simulink model "plant_neural"  (R2020a)
settings: Solver=VariableStepAuto  StartTime=0.0  StopTime=200  RelTol=1e-3
values from neighbouring files (symbols this model uses):
  Ca = 0.005    [reproduce_examples.m]
  Cb = 0.005    [reproduce_examples.m]
  dt = 0.05    [reproduce_examples.m]
  fA = 2    [reproduce_examples.m]
  fB = 2    [reproduce_examples.m]
  V = 3    [reproduce_examples.m]
libraries: simulink x2, neural x1
settings Model: Creator=salvatore  LastModifiedBy=salvatore
settings DataIOCC: ExternalInput=Fb  FinalStateName=p  SaveFormat=Array  SignalLogging=off  OutputSaveName=pH, valve
settings DebuggingCC: UnderSpecifiedDimensionMsg=warning

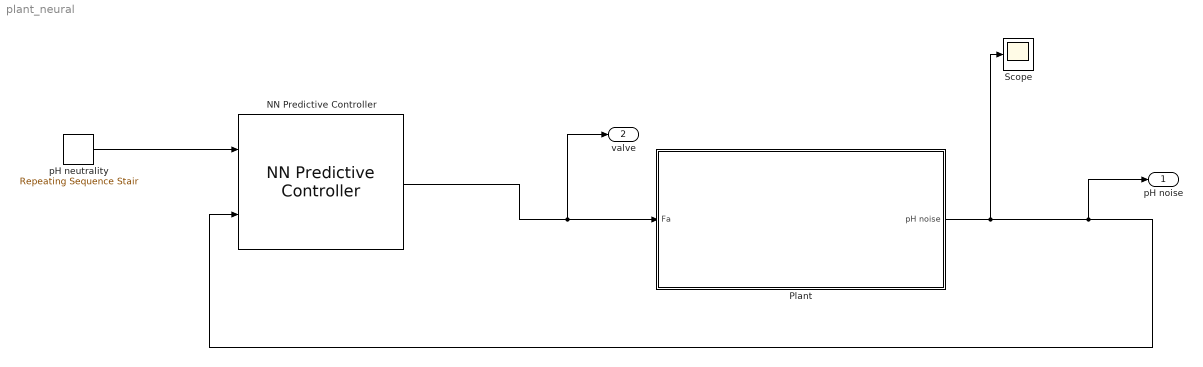
== system plant_neural ==
  NN Predictive Controller : neural/Control Systems/NN Predictive Controller  epochs=3000  minp=49.141375352717240332  maxp=50.989811034304850068  mint=4.3097489678251754697  maxt=50.989811034304850068  Normalize=0  IW=[-0.93780239581817526062 -0.66326789240486860866 -1.2871031244271990968;1.9683728574995722482 1.0271333939241629185 0.44317348386700522456;0.75017590865152150581 -1.0780019808511700496 1.0869414820155824941;1.4559030881353915987 -0.12800319720607680751 0.95276790366173158553;18.087212465487294111 -2.91864184413527461 -14.566729179573659536;1.2400378014953861161 0.1375233693964867665 0.77502847574575350897;0.33253977855035904421 1.7304982921477456426 1.3544701109704289088;0.64182775575216644004 1.4117570112710189356 -0.65500462374746837302;1.0980139843273326594 1.4813102838210283618 -1.1355980615640355325;-1.8940112774775548221 -1.0242663724758558352 -1.1299048301245802062;1.855202007600092351 0.12165935101839298049 -0.79891607712896228755;-0.32930667884939862633 -1.5538501135001399067 -0.75067226960660971002;-1.072431998622664695 0.65403235548163929369 1.0984496057562562754;0.81019484569678412722 0.33526087379087021745 -1.5256456319409121836;-1.4522827265983397904 1.485812570700000057 0.37966236721378082697;-1.1923047419461934027 1.5162107446574706326 -1.0145022129936238642;0.30440125275836227292 1.3381364521867997741 1.0876416367064514201;-0.92200869750636560429 -0.32060881750568615001 -1.2246860483548469567;-0.60210950948219532641 -1.4986276837771175252 -0.080409026582326029176;-0.403355788115020375 0.24290872576269775807 2.3590303610904217457;-0.19706504822617046391 -1.023417972628119843 -0.52486522394001777769;-0.3686768376053149443 -0.88079531358954077369 -1.5303785213897103112;0.53120649011313425536 -0.82254467800489938778 -1.3528928606977603799;-1.2733849000756418679 -1.6495155478202192523 -0.39519231325363640694;-1.302693854262735762 1.0188200785665699755 -0.7030027146678801131;-1.3444294028268313212 0.92366281600611421787 -0.89920403196537579404;-0.71934229537864724513 0.098840184553247473209 1.9183675969502649306;1.1859515817055199527 -0.72039123611880495623 0.80635457452268266554;-0.91328157335381698889 1.1116547471258793056 1.5977262904151019463;0.88358410119703434393 0.18945012830566010376 -0.20403044228299269114;0.68771194682422021049 1.5767992308421543424 1.5215138710997695437;1.1746781130618693112 1.3205123690215239129 -1.7492648228398455235;1.366694751554343723 -0.59956811717985569743 0.46771085416193147744;-0.76196806167879460592 0.11135710623432852617 1.1872906506293119389;-0.63585738589058671266 -0.51021415961426375141 -0.93569241318754825532;0.15302930875759376828 0.38592558000686749686 1.4065606172366182935;-1.0258043101484959347 1.6494109276893627047 1.4700854999973029802;1.1035774350367175689 0.78663020300303343468 1.0269086353427672176;1.0614598671358197457 -1.2948141427555899252 0.25657285536884832933;0.048561450203500375333 1.1539886836612518461 1.0587047076348954366]  LW1_2=[-0.62041762781086506884 -1.2878921055441192589 1.3341064249686134247;-0.4452363508536192338 0.41776855322875938725 -0.16173792171746106949;0.7856277323655095346 -1.4328813778630613562 -1.4048068556256605444;-1.1026662378935343511 -0.13613422789046639161 -1.582104961796532594;9.2826822808918620922 -15.216546321325413516 1.746026347965279113;-0.89963594778431121846 -1.5624571017304575982 -1.1696900531712195459;-1.0380744821846603632 0.80818670706969764073 -0.28584295651548530248;-2.0100154521868383029 -2.7516072687074384362 1.5959436752205937715;1.1440492783128197729 0.83935914794030452857 0.13137238494993638827;-0.17328463839084443099 -0.30390637859945579535 -0.51995736605186482215;-0.54032173048821574568 -0.38414956417682477596 -1.3561814656743973462;-1.0874881996895870984 -1.5564886858033175621 -0.19773337940546048541;1.1710921340230626697 -1.0606306130658302855 1.1424339619712420291;-0.34790852481674128249 -1.3671355131979634479 -1.2360864438805858612;1.4392017742796474611 0.38518544750179245506 -0.12885364617398359366;0.41412038455630650891 -0.79867140581223539098 1.0466562009230124808;-0.42970303418967958908 1.0765221590345304126 -1.4956312828675100146;1.4379506574267850727 1.2978382988600296599 0.67962005247037582389;0.89538010453812910683 1.276425240546694706 1.3508334040361238415;-0.16637092117171603523 0.0048575864307608667553 -0.95787243818502754156;1.0941255058475363171 -1.2496437309479786482 -1.6035705320276094632;1.4249238601570537455 -0.95316005127912184491 0.63714090417240143438;-0.32080390345351345038 0.16230007420602191037 1.9459977888606936336;-0.66671428962549628139 1.134168699749920517 0.55528982774655066823;0.39914983905510748041 -0.60645365770087922286 1.7410306582268146869;1.369987504183791005 -0.17140586938442378684 -1.1112576424741043013;0.88535442154446764018 0.59339915818222865873 1.1636166105827401296;-0.51693099978261292105 1.8481114067055248729 -0.64860148033353415276;0.86149168240209295089 -1.1144179111944447769 -0.29601512276503749721;1.8168695740521629833 0.9606138608186394201 -1.2248969681246073549;0.18613707562859144184 0.31093738389837610736 1.1586827272944042466;0.18384056074634250177 -0.06569561361777594144 0.53337760519972754469;-0.79892203697135377727 1.6575502283018046512 0.97902857163499057425;-1.7227854292604303232 -0.46185913158445146554 1.2421345908758245624;-1.1699157231057202289 -1.1656192475389974827 -1.5771178680323889587;-1.3992694065135036219 0.36304775877899103653 1.551469629702085351;-0.19023048985576973546 0.7495605338521728056 0.036042435367489758513;-1.5862432648658111312 -0.51387741920938923013 0.93417374728402524653;1.4268590699500380836 1.0441978897072439203 0.83533526411353720142;0.47269246211427085047 1.4569527321962194577 0.90941043120806075439]  LW2_1=[-0.66653421186476879967 -2.3712304948727283005 0.11942670348945146064 0.30208230055944201853 -0.15692778228640197336 -0.35950126395863518658 0.09773454763742397966 -0.41867824898828193136 0.5537078005106340628 0.36924865693212843842 -0.38671729588311865022 0.38461463905337617275 0.47125947419330549426 -0.71456955098225838352 0.10753548983805111261 -0.3776052745659378429 0.14761236314075976139 0.41525079704560979854 -0.95160198566457088187 0.679186802666668199 0.244621722809567399 -0.27327517649929583543 -0.1999592102286981421 -0.027090443201696387532 0.22999930288450973204 -0.043644044702432986671 0.59475549883440670396 0.08020888099440409702 -0.062075004625083300691 0.69916082819646241386 0.1573521172310034244 0.31863025260330235522 -0.19631262295613918778 0.51685318417522729817 -0.046828393152410316413 1.2045935795346516262 -0.47849157362152594519 0.68975629544934580206 0.074856560607579905597 -0.42847594362385321709]  B1=[2.5672464899590048404;-170.64449277703008079;-2.1630320896469008574;2.1661759738817525367;0.20955525796052568155;1.907413289370134768;1.7537648794198914537;1.7570397648592248618;-1.510171361480447727;1.4335841467054168952;1.3768291617565806551;1.1078535178173269937;-1.0630899555232686815;0.90212784634881437729;-0.72050608555673145705;-0.60937469228950069677;0.50924077145348967122;-0.35642750821878815826;-0.10173522078065622143;0.01835621770530715402;0.19928770939365009207;0.15113090330299616681;-0.33623361906458620885;-0.52256622681785103168;0.56334603835885599388;0.72066291768343948565;0.81010159705356599158;-1.0160798924089358142;1.0839109593114522045;1.120367655511463223;1.3436935869649371256;1.4163930936675419581;-1.653743695745887532;-1.7655981945075955863;-1.9161927166153283064;-2.0411231849379389836;-2.193559035776065258;-2.3669642277819522569;2.4565641560167699176;2.752801679695834558]  B2=0.84267571160203313951  max_i_int=100  min_i_int=2  limit_output=1  max_output=14  min_output=0  Use_Previous_Weights=1  N2=11  Nu=2  Ts=1  rho=0.001  alpha=0.001  csrchfun=csrchbac  maxiter=2  S1=40  Ni=3  Nj=3  sim_file=plant  trainfun=trainlm  Use_validation=1  Use_Testing=1  max_i=51  min_i=49  sam_training=2000
      settings: SourceProductBaseCode=NN
  Plant : Subsystem
  Scope : Scope
  pH neutrality : simulink/Sources/Repeating Sequence Stair  OutValues=reference  tsamp=time_ref  OutMin=[]  OutMax=[]  OutDataTypeStr=double  OutputDataTypeScalingMode=double  OutDataType=fixdt(0,8)  ConRadixGroup=Best Precision: Vector-wise  OutScaling=2^-12
  pH noise : Outport  SignalName=ph_noise
  valve : Outport  Port=2  SignalName=valve
  wires:
  NN Predictive Controller/1 -> valve/1, Plant/1(Fa)
  Plant/1(pH noise) -> Scope/1, NN Predictive Controller/2, pH noise/1
  pH neutrality/1 -> NN Predictive Controller/1

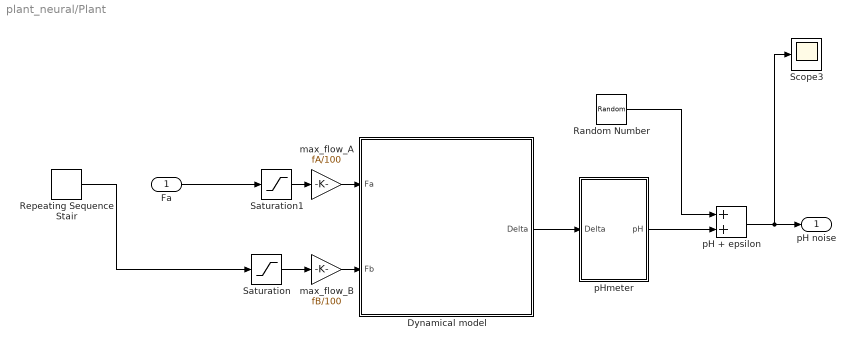
== system plant_neural/Plant ==
  Fa : Inport
  Dynamical model : Subsystem
  Random Number : RandomNumber  Variance=0.01  SampleTime=dt
  Repeating Sequence Stair : simulink/Sources/Repeating Sequence Stair  OutValues=out_valv  tsamp=time_valv  OutMin=[]  OutMax=[]  OutDataTypeStr=double  OutputDataTypeScalingMode=double  OutDataType=fixdt(0,8)  ConRadixGroup=Best Precision: Vector-wise  OutScaling=2^-12
  Saturation : Saturate  UpperLimit=100  LowerLimit=0
  Saturation1 : Saturate  UpperLimit=100  LowerLimit=0
  Scope3 : Scope
  max_flow_A : Gain  Gain=fA/100
  max_flow_B : Gain  Gain=fB/100
  pH + epsilon : Sum
  pHmeter : Subsystem
  pH noise : Outport
  wires:
  max_flow_A/1 -> Dynamical model/1(Fa)
  max_flow_B/1 -> Dynamical model/2(Fb)
  pH + epsilon/1 -> Scope3/1, pH noise/1
  pHmeter/1(pH) -> pH + epsilon/2
  Saturation1/1 -> max_flow_A/1
  Random Number/1 -> pH + epsilon/1
  Saturation/1 -> max_flow_B/1
  Dynamical model/1(Delta) -> pHmeter/1(Delta)
  Fa/1 -> Saturation1/1
  Repeating Sequence Stair/1 -> Saturation/1

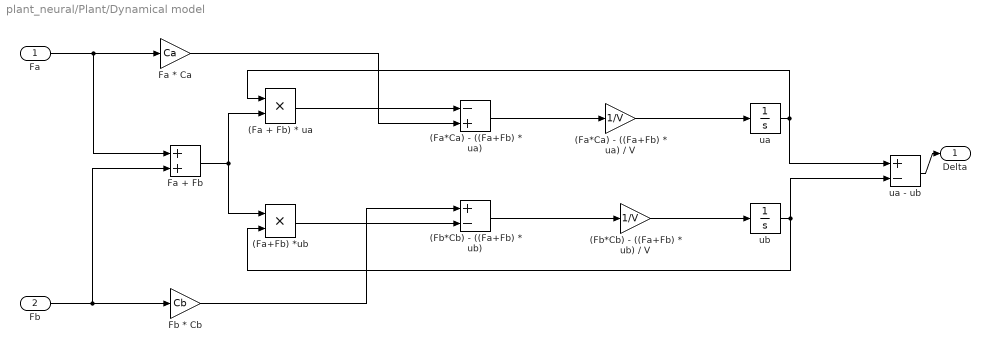
== system plant_neural/Plant/Dynamical model ==
  Fa : Inport
  Fb : Inport  Port=2
  "(Fa + Fb) * ua " : Product  Inputs=**
  (Fa*Ca) - ((Fa+Fb) * ua) : Sum  Inputs=-+
  (Fa*Ca) - ((Fa+Fb) * ua) / V : Gain  Gain=1/V
  "(Fa+Fb) *ub  " : Product  Inputs=**
  (Fb*Cb) - ((Fa+Fb) * ub) : Sum  Inputs=+-
  (Fb*Cb) - ((Fa+Fb) * ub) / V : Gain  Gain=1/V
  "Fa * Ca " : Gain  Gain=Ca
  Fa + Fb : Sum
  Fb * Cb : Gain  Gain=Cb
  ua : Integrator  LimitOutput=on  UpperSaturationLimit=1  LowerSaturationLimit=0
  ua - ub : Sum  Inputs=+-
  ub : Integrator  LimitOutput=on  UpperSaturationLimit=1  LowerSaturationLimit=0
  Delta : Outport
  wires:
  (Fa*Ca) - ((Fa+Fb) * ua) / V/1 -> ua/1
  Fa/1 -> Fa + Fb/1, "Fa * Ca "/1
  "(Fa + Fb) * ua "/1 -> (Fa*Ca) - ((Fa+Fb) * ua)/1
  "Fa * Ca "/1 -> (Fa*Ca) - ((Fa+Fb) * ua)/2
  ub/1 -> ua - ub/2, "(Fa+Fb) *ub  "/2
  Fb/1 -> Fa + Fb/2, Fb * Cb/1
  Fb * Cb/1 -> (Fb*Cb) - ((Fa+Fb) * ub)/1
  "(Fa+Fb) *ub  "/1 -> (Fb*Cb) - ((Fa+Fb) * ub)/2
  Fa + Fb/1 -> "(Fa+Fb) *ub  "/1, "(Fa + Fb) * ua "/2
  (Fb*Cb) - ((Fa+Fb) * ub) / V/1 -> ub/1
  ua - ub/1 -> Delta/1
  ua/1 -> ua - ub/1, "(Fa + Fb) * ua "/1
  (Fa*Ca) - ((Fa+Fb) * ua)/1 -> (Fa*Ca) - ((Fa+Fb) * ua) / V/1
  (Fb*Cb) - ((Fa+Fb) * ub)/1 -> (Fb*Cb) - ((Fa+Fb) * ub) / V/1

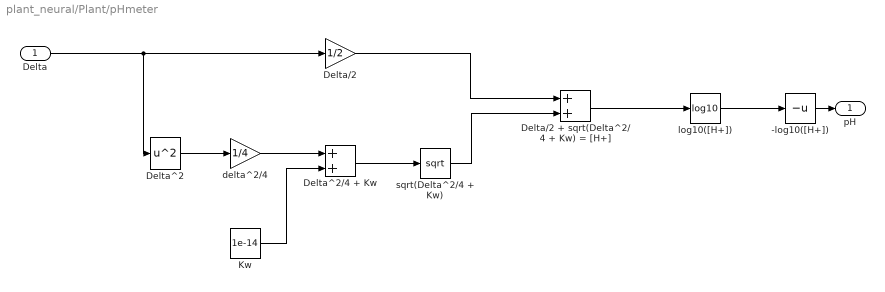
== system plant_neural/Plant/pHmeter ==
  Delta : Inport
  -log10([H+]) : UnaryMinus
  Delta/2 : Gain  Gain=1/2
  Delta/2 + sqrt(Delta^2/4 + Kw) = [H+] : Sum
  Delta^2 : Math  Operator=square  SaturateOnIntegerOverflow=on
  Delta^2/4 + Kw : Sum
  Kw : Constant  Value=1e-14
  delta^2/4 : Gain  Gain=1/4
  "log10([H+]) " : Math  Operator=log10  SaturateOnIntegerOverflow=on
  sqrt(Delta^2/4 + Kw) : Sqrt  SaturateOnIntegerOverflow=on
  pH : Outport
  wires:
  "log10([H+]) "/1 -> -log10([H+])/1
  Delta^2/4 + Kw/1 -> sqrt(Delta^2/4 + Kw)/1
  -log10([H+])/1 -> pH/1
  Kw/1 -> Delta^2/4 + Kw/2
  sqrt(Delta^2/4 + Kw)/1 -> Delta/2 + sqrt(Delta^2/4 + Kw) = [H+]/2
  Delta/2 + sqrt(Delta^2/4 + Kw) = [H+]/1 -> "log10([H+]) "/1
  Delta/1 -> Delta/2/1, Delta^2/1
  Delta^2/1 -> delta^2/4/1
  delta^2/4/1 -> Delta^2/4 + Kw/1
  Delta/2/1 -> Delta/2 + sqrt(Delta^2/4 + Kw) = [H+]/1
